simulink model "zirco"  (R2013a)
settings: Solver=ode4  StartTime=0.0  StopTime=1  FixedStep=10^-5  RelTol=1e-3
libraries: simulink x1
settings Model: Creator=Eren  LastModifiedBy=Eren

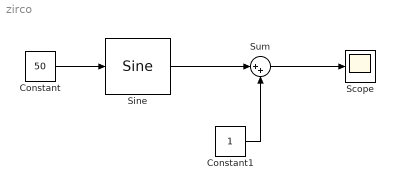
== system zirco ==
  Constant : Constant  Value=50
  Constant1 : Constant
  Scope : Scope
  Sine : simulink/Lookup Tables/Sine  Formula=sin(2*pi*u)  NumDataPoints=(2^5)+1  OutputWordLength=16
  Sum : Sum  Inputs=|++
  wires:
  Constant1/1 -> Sum/2
  Sine/1 -> Sum/1
  Constant/1 -> Sine/1
  Sum/1 -> Scope/1
